simulink model "JIerro13"  (R2021a)
settings: Solver=VariableStepAuto  StartTime=0.0  StopTime=10.0  RelTol=1e-3
libraries: simulink x3
settings Model: Creator=O1  LastModifiedBy=O1

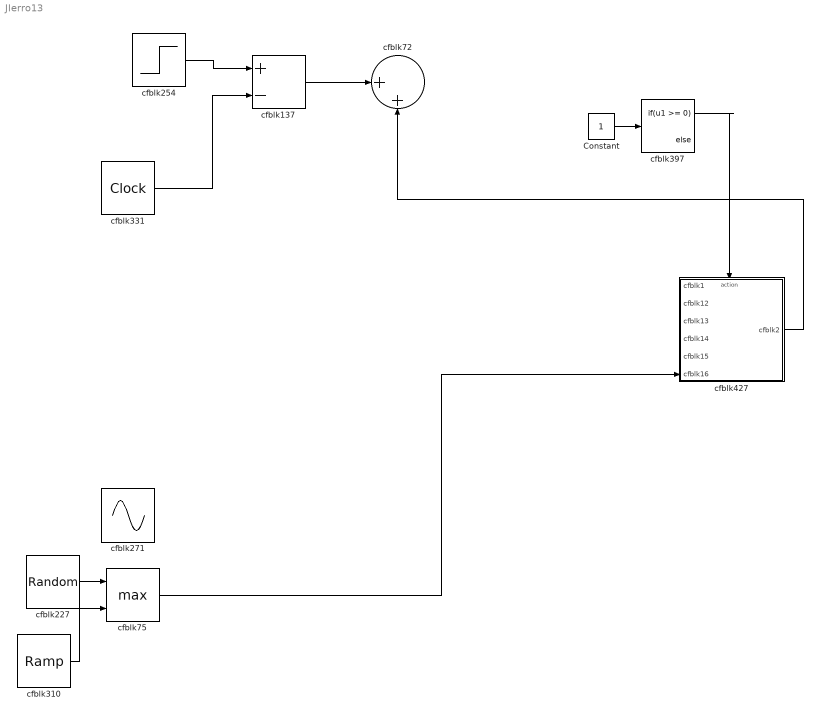
== system JIerro13 ==
  Constant : Constant
  cfblk137 : Sum  Inputs=+-
  cfblk227 : RandomNumber  Mean=[-34488.154122]  Variance=[75351.385843]  Seed=[84700931.000000]  SampleTime=0.1
  cfblk254 : Step  Time=[2.000000]  Before=[801221138.121829]  After=[-89823733.021611]  SampleTime=0
  cfblk271 : Sin  Amplitude=[-921373321.042865]  Bias=[632755603.310922]  SampleTime=0
  cfblk310 : simulink/Sources/Ramp  slope=[3689.412226]  start=[46.253601]  InitialOutput=[-250282.865254]
  cfblk331 : DigitalClock
  cfblk397 : If  IfExpression=u1 >= 0  SampleTime=1
  cfblk427 : Subsystem  TreatAsAtomicUnit=on
  cfblk72 : Sum  Inputs=|++
  cfblk75 : MinMax  Function=max  Inputs=2
  wires:
  cfblk427/1(cfblk2) -> cfblk72/2
  cfblk75/1 -> cfblk427/6(cfblk16)
  cfblk227/1 -> cfblk75/1
  Constant/1 -> cfblk397/1
  cfblk397/1 -> cfblk427/Action
  cfblk254/1 -> cfblk137/1
  cfblk137/1 -> cfblk72/1
  cfblk310/1 -> cfblk75/2
  cfblk331/1 -> cfblk137/2

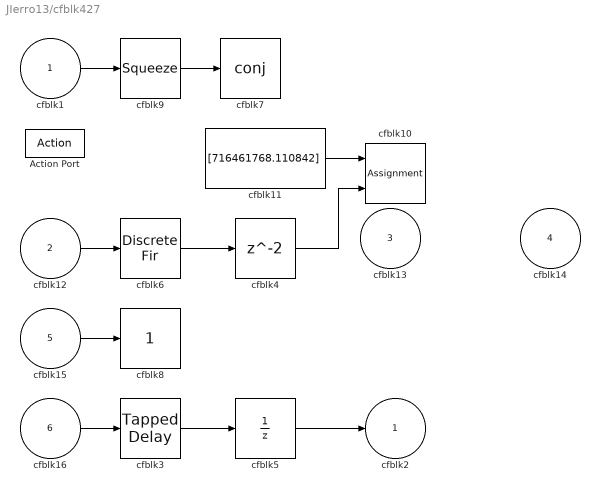
== system JIerro13/cfblk427 ==
  cfblk1 : Inport
  cfblk12 : Inport  Port=2
  cfblk13 : Inport  Port=3
  cfblk14 : Inport  Port=4
  cfblk15 : Inport  Port=5
  cfblk16 : Inport  Port=6
  Action Port : ActionPort  ActionPortLabel=if(u1 >= 0)
  cfblk10 : Assignment  DiagnosticForDimensions=Warning  IndexOptions=Index vector (dialog)  Indices=1  OutputSizes=1
  cfblk11 : Constant  Value=[716461768.110842]  SampleTime=1
  cfblk3 : simulink/Discrete/Tapped Delay  vinit=0.0  samptime=-1  NumDelays=1  DelayOrder=Oldest  includeCurrent=off
  cfblk4 : Delay
  cfblk5 : UnitDelay  SampleTime=-1  HasFrameUpgradeWarning=on
  cfblk6 : DiscreteFir
  cfblk7 : Math  Operator=conj  SaturateOnIntegerOverflow=on
  cfblk8 : simulink/Math Operations/Slider Gain  gain=1  low=0  high=2
  cfblk9 : Squeeze
  cfblk2 : Outport
  wires:
  cfblk15/1 -> cfblk8/1
  cfblk4/1 -> cfblk10/2
  cfblk11/1 -> cfblk10/1
  cfblk3/1 -> cfblk5/1
  cfblk5/1 -> cfblk2/1
  cfblk12/1 -> cfblk6/1
  cfblk16/1 -> cfblk3/1
  cfblk1/1 -> cfblk9/1
  cfblk6/1 -> cfblk4/1
  cfblk9/1 -> cfblk7/1
